simulink model "PD_Controller_mod"  (R2019b)
settings: Solver=VariableStepAuto  StartTime=0.0  StopTime=10  RelTol=1e-3
StopFcn:
  | Colors=hsv(5)';
  | for i=1:5
  | plot(out.tout,out.R_PD(:,i),'color',Colors(:,i),'LineWidth',1.5)
  | hold on
  | end
  | grid on
  | legend('Joint1','Joint2','Joint3','Joint4','Joint5')
  | title(['Response Vs Input of Joints Via PD Controller'])
  | xlabel('Time')
  | ylabel('Response')
libraries: simulink x5
(part 1 of 3)
settings Model: Creator=baran  LastModifiedBy=baran

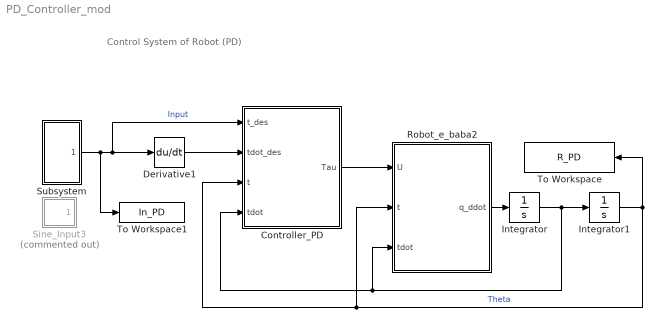
== system PD_Controller_mod ==
  note: Control System of Robot (PD)
  Controller_PD : MATLAB Function  TreatAsAtomicUnit=on
  Derivative1 : Derivative
  Integrator : Integrator  InitialCondition=[0 0 0 0 0]'
  Integrator1 : Integrator  InitialCondition=[-5 -4 -3 -2 -1]'
  Robot_e_baba2 : MATLAB Function  TreatAsAtomicUnit=on
  Sine_Input3 : Subsystem  Commented=on
  Subsystem : Subsystem
  To Workspace : ToWorkspace  VariableName=R_PD  SampleTime=-1
  To Workspace1 : ToWorkspace  VariableName=In_PD  SampleTime=-1
  wires:
  Integrator/1 -> Controller_PD/4(tdot), Robot_e_baba2/3(tdot), Integrator1/1
  Robot_e_baba2/1(q_ddot) -> Integrator/1
  Integrator1/1 -> To Workspace/1, Controller_PD/3(t), Robot_e_baba2/2(t)  "Theta"
  Controller_PD/1(Tau) -> Robot_e_baba2/1(U)
  Derivative1/1 -> Controller_PD/2(tdot_des)
  Subsystem/1(INPUT) -> Controller_PD/1(t_des), Derivative1/1, To Workspace1/1  "Input"

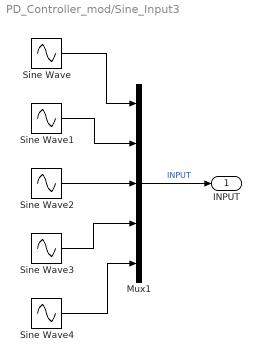
== system PD_Controller_mod/Sine_Input3 ==
  Mux1 : Mux  Inputs=5
  Sine Wave : Sin  Bias=2  Frequency=0.5  SampleTime=0
  Sine Wave1 : Sin  Bias=3  Frequency=4  SampleTime=0
  Sine Wave2 : Sin  Amplitude=2  SampleTime=0
  Sine Wave3 : Sin  Amplitude=2  SampleTime=0
  Sine Wave4 : Sin  Amplitude=2  SampleTime=0
  INPUT : Outport
  wires:
  Sine Wave3/1 -> Mux1/4
  Sine Wave4/1 -> Mux1/5
  Sine Wave/1 -> Mux1/1
  Sine Wave1/1 -> Mux1/2
  Mux1/1 -> INPUT/1  "INPUT"
  Sine Wave2/1 -> Mux1/3

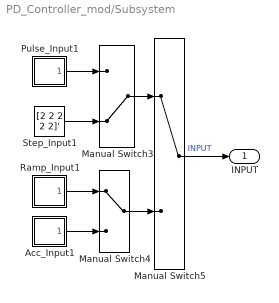
== system PD_Controller_mod/Subsystem ==
  Acc_Input1 : Subsystem
  Manual Switch3 : ManualSwitch  CurrentSetting=0
  Manual Switch4 : ManualSwitch
  Manual Switch5 : ManualSwitch
  Pulse_Input1 : Subsystem
  Ramp_Input1 : Subsystem
  Step_Input1 : Constant  Value=[2 2 2 2 2]'
  INPUT : Outport
  wires:
  Step_Input1/1 -> Manual Switch3/2
  Manual Switch3/1 -> Manual Switch5/1
  Ramp_Input1/1(INPUT) -> Manual Switch4/1
  Pulse_Input1/1(INPUT) -> Manual Switch3/1
  Manual Switch4/1 -> Manual Switch5/2
  Acc_Input1/1(INPUT) -> Manual Switch4/2
  Manual Switch5/1 -> INPUT/1  "INPUT"

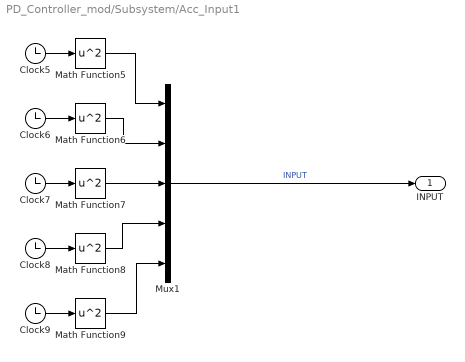
== system PD_Controller_mod/Subsystem/Acc_Input1 ==
  Clock{5..9} (5 alike) : Clock
  Math Function{5..9} (5 alike) : Math  Operator=square  SignedPower=off  SaturateOnIntegerOverflow=on
  Mux1 : Mux  Inputs=5
  INPUT : Outport
  wires:
  Math Function8/1 -> Mux1/4
  Math Function9/1 -> Mux1/5
  Clock5/1 -> Math Function5/1
  Math Function7/1 -> Mux1/3
  Clock9/1 -> Math Function9/1
  Math Function6/1 -> Mux1/2
  Clock8/1 -> Math Function8/1
  Clock7/1 -> Math Function7/1
  Math Function5/1 -> Mux1/1
  Clock6/1 -> Math Function6/1
  Mux1/1 -> INPUT/1  "INPUT"

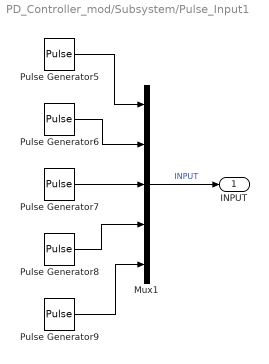
== system PD_Controller_mod/Subsystem/Pulse_Input1 ==
  Mux1 : Mux  Inputs=5
  Pulse Generator5 : DiscretePulseGenerator  PulseType=Time based  Period=10  PulseWidth=0.1
  Pulse Generator6 : DiscretePulseGenerator  PulseType=Time based  Amplitude=0.5  Period=10  PulseWidth=0.1
  Pulse Generator7 : DiscretePulseGenerator  PulseType=Time based  Amplitude=0.25  Period=10  PulseWidth=0.1
  Pulse Generator8 : DiscretePulseGenerator  PulseType=Time based  Amplitude=0.1  Period=10  PulseWidth=0.1
  Pulse Generator9 : DiscretePulseGenerator  PulseType=Time based  Amplitude=0.7  Period=10  PulseWidth=0.1
  INPUT : Outport
  wires:
  Pulse Generator7/1 -> Mux1/3
  Mux1/1 -> INPUT/1  "INPUT"
  Pulse Generator6/1 -> Mux1/2
  Pulse Generator5/1 -> Mux1/1
  Pulse Generator9/1 -> Mux1/5
  Pulse Generator8/1 -> Mux1/4

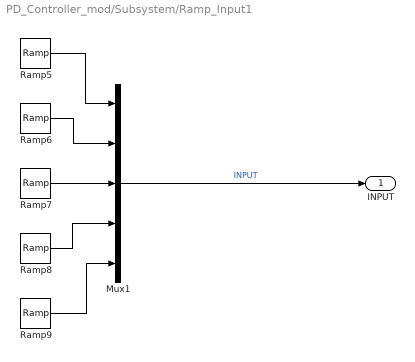
== system PD_Controller_mod/Subsystem/Ramp_Input1 ==
  Mux1 : Mux  Inputs=5
  Ramp{5..9} (5 alike) : simulink/Sources/Ramp  slope=2  start=0.0001  InitialOutput=0
  INPUT : Outport
  wires:
  Ramp5/1 -> Mux1/1
  Ramp6/1 -> Mux1/2
  Ramp8/1 -> Mux1/4
  Ramp7/1 -> Mux1/3
  Ramp9/1 -> Mux1/5
  Mux1/1 -> INPUT/1  "INPUT"
